simulink model "Lab1_1"  (R2018a)
settings: Solver=VariableStepAuto  StartTime=0.0  StopTime=10.0  RelTol=1e-9
settings Model: Creator=melab2  LastModifiedBy=melab2

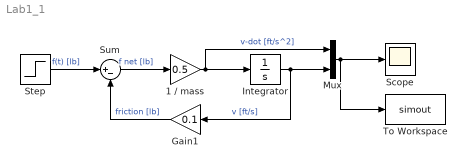
== system Lab1_1 ==
  1 / mass : Gain  Gain=0.5
  Gain1 : Gain  Gain=0.1
  "Integrator " : Integrator
  Mux : Mux  Inputs=2
  "Scope " : Scope
  "Step " : Step  SampleTime=0
  Sum : Sum  Inputs=|+-
  "To Workspace " : ToWorkspace  VariableName=simout  SampleTime=-1
  wires:
  "Step "/1 -> Sum/1  "f(t) [lb]"
  Sum/1 -> 1 / mass/1  "f net [lb]"
  1 / mass/1 -> Mux/1, "Integrator "/1  "v-dot [ft/s^2]"
  Gain1/1 -> Sum/2  "friction [lb]"
  "Integrator "/1 -> Gain1/1, Mux/2  "v [ft/s]"
  Mux/1 -> "To Workspace "/1, "Scope "/1
